simulink model "sgMdl_IO682_ARINC429Loopback"  (R2024b)
settings: Solver=FixedStepAuto  StartTime=0.0  StopTime=inf  RelTol=1e-3  EnableMultiTasking=on
undefined symbols (not defined in the file): IO682
libraries: speedgoatlib_IO682 x9
Description:
  | IO682 - ARINC 429 Loopback
settings Model: ModifiedByFormat=Speedgoat  SimulationMode=external  ExtModeTrigDuration=100000  Creator=Speedgoat  LastModifiedBy=Speedgoat
settings SolverCC: ConcurrentTasks=on  AlgebraicLoopSolver=TrustRegion  PositivePriorityOrder=on
settings DataIOCC: LimitDataPoints=on  SaveFormat=Array  ReturnWorkspaceOutputs=off
settings OptimizationCC: BlockReduction=off  OptimizeBlockIOStorage=off  BufferReuse=off  GlobalBufferReuse=off  ExpressionFolding=off  LocalBlockOutputs=off  OptimizeDataStoreBuffers=off  BusAssignmentInplaceUpdate=off
settings DebuggingCC: SolverPrmCheckMsg=warning  TasksWithSamePriorityMsg=none  UnconnectedInputMsg=warning  UnconnectedOutputMsg=warning  UnconnectedLineMsg=warning  AllowSymbolicDim=off  SFUnexpectedBacktrackingDiag=warning  SFNoUnconditionalDefaultTransitionDiag=warning  SFExecutionAtInitializationDiag=none  ArithmeticOperatorsInVariantConditions=warning
settings HardwareCC: ProdBitPerLong=64  ProdLongLongMode=on  ProdHWDeviceType=Intel->x86-64 (Linux 64)
settings ModelReferenceCC: EnableRefExpFcnMdlSchedulingChecks=on  PropagateSignalLabelsOutOfModel=off
settings SFSimCC: SimUseLocalCustomCode=off  CustomCodeUndefinedFunction=UseInterfaceOnly
settings RTWCC: Description=Speedgoat Real-Time Target Machine  SystemTargetFile=speedgoat.tlc  TemplateMakefile=slrealtime_default_tmf  RTWUseLocalCustomCode=off  Toolchain=Simulink Real-Time Toolchain  BuildConfiguration=Faster Runs  TargetLang=C++  GPUComputeCapability=3.5  DLArmComputeVersion=19.05
settings CodeAppCC: StateflowObjectComments=on
settings SimulinkRealTimeTargetCC: SubcomponentCodeInterfacePackaging=Reusable function  InstructionSetFMA=off  LogToMDFFile=off  SLRTFileLogMaxRuns=10  UseGCCFastMath=on
settings ConfigComp: CovMetricSettings=dw  CovSaveCumulativeToWorkspaceVar=on  CovSaveSingleToWorkspaceVar=on  CovExternalEMLEnable=off  CovSFcnEnable=off  CovBoundaryAbsTol=1.0e-5

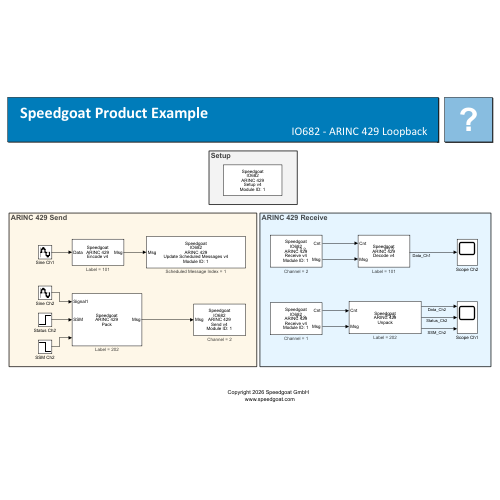
[thumbnail: Simulink's stored preview of the top-level diagram]
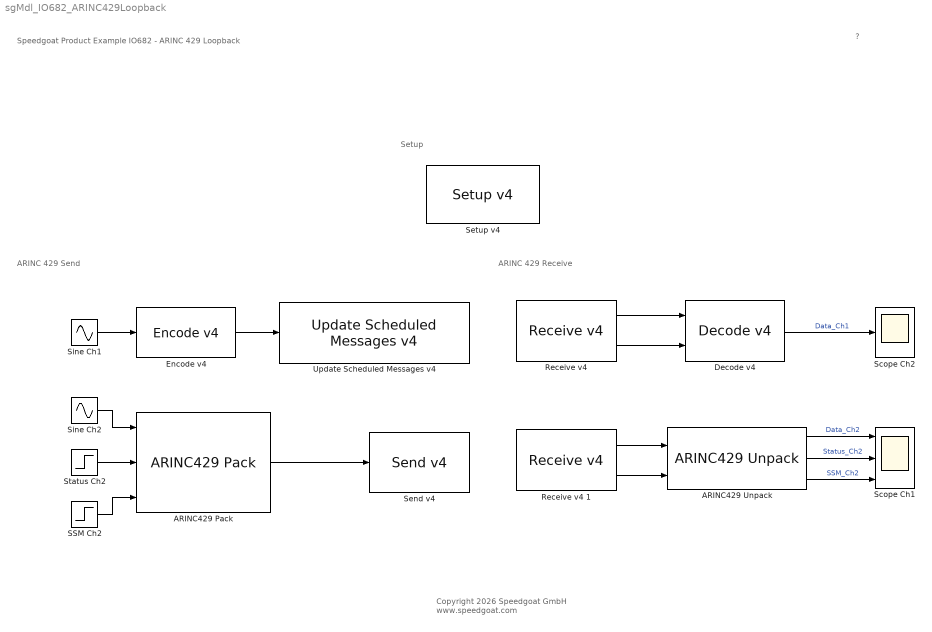
== system sgMdl_IO682_ARINC429Loopback ==
  note: ARINC 429 Send
  note: ARINC 429 Receive
  note: Setup
  note: Speedgoat Product Example
      | IO682 - ARINC 429 Loopback
  note: ?
  note: Copyright 2026 Speedgoat GmbH
      |  www.speedgoat.com
  "ARINC429 Pack " : speedgoatlib_IO682/ARINC429 Pack   parLabel=202  parSdi=2  parSsm=3  parSignals={ 'Sine', '11', '18', 'BNR', '10', '0', '-Inf', 'Inf', 'on'; 'Status Bit', '29', '1', 'DSC', '1', '0', '-Inf', 'Inf', 'off'; 'SSM', '30', '2', 'SSM', '1', '0', '-Inf', 'Inf', 'off' }
      settings: AttributesFormatString=Label = %<parLabel>  SourceProductName=IO682
  "ARINC429 Unpack " : speedgoatlib_IO682/ARINC429 Unpack   parLabel=202  parSdi=2  parSignals={ 'Sine', '11', '18', 'BNR', '10', '0', '-Inf', 'Inf', 'on'; 'Status Bit', '29', '1', 'DSC', '1', '0', '-Inf', 'Inf', 'off'; 'SSM', '30', '2', 'SSM', '1', '0', '-Inf', 'Inf', 'off' }  parEnTimeTag=off  parEnStatus=off  parEnRaw=off
      settings: AttributesFormatString=Label = %<parLabel>  SourceProductName=IO682
  "Decode v4 " : speedgoatlib_IO682/Decode v4   parLabel=101  parDataType=BNR  parResolution=10  parSdi=-1  parEnSDIBits=off  parHoldLastVal=on  parLabelOutput=off  parSSMOutput=off  parTimeTags=off  parStatus=off
      settings: AttributesFormatString=Label = %<parLabel>  SourceProductName=IO682
  "Encode v4 " : speedgoatlib_IO682/Encode v4   parLabel=101  parDataType=BNR  parResolution=10  parBits=19  parSdi=-1  parSsm=3  parEnSDIBits=off  parEnSSM=off
      settings: AttributesFormatString=Label = %<parLabel>  SourceProductName=IO682
  "Receive v4 " : speedgoatlib_IO682/Receive v4   parModuleId=1  parChannel=2  parMaxWords=50  parSampleTime=0.05  parEnTimeTags=off
      settings: AttributesFormatString=Channel = %<parChannel>  SourceProductName=IO682
  Receive v4 1 : speedgoatlib_IO682/Receive v4   parModuleId=1  parChannel=1  parMaxWords=50  parSampleTime=0.005  parEnTimeTags=off
      settings: AttributesFormatString=Channel = %<parChannel>  SourceProductName=IO682
  SSM Ch2 : Step  Time=5  Before=3  After=0  SampleTime=0
  Scope Ch1 : Scope  NumInputPorts=3
  Scope Ch2 : Scope
  "Send v4 " : speedgoatlib_IO682/Send v4   parModuleId=1  parChannel=2  parSampleTime=-1  parTxCtrl=off
      settings: AttributesFormatString=Channel = %<parChannel>  SourceProductName=IO682
  "Setup v4 " : speedgoatlib_IO682/Setup v4   parModuleId=1  parBoardVariant=IO682-8-8  parPciSlot=-1  parChannelMode=Manual  parInBitRate1=100000  parInBufferMode1=Individual  parInEnable1=on  parInParity1=on  parInInternalWrap1=off  parInBitRate2=100000  parInBufferMode2=Individual  parInEnable2=on  parInParity2=on  parInInternalWrap2=off  parInBitRate3=100000  parInBufferMode3=Individual  parInEnable3=on  parInParity3=on  parInInternalWrap3=off  parInBitRate4=100000  parInBufferMode4=Individual  parInEnable4=on  parInParity4=on  parInInternalWrap4=off  parInBitRate5=100000  parInBufferMode5=Individual  parInEnable5=off  parInParity5=on  parInInternalWrap5=off  parInBitRate6=100000  parInBufferMode6=Individual  parInEnable6=off  parInParity6=on  parInInternalWrap6=off  parInBitRate7=100000  parInBufferMode7=Individual  parInEnable7=off  parInParity7=on  parInInternalWrap7=off  parInBitRate8=100000  parInBufferMode8=Individual  parInEnable8=off  parInParity8=on  parInInternalWrap8=off  parInBitRate9=100000  parInBufferMode9=Individual  parInEnable9=on  parInParity9=on  parInInternalWrap9=off  parInBitRate10=100000  parInBufferMode10=Individual  parInEnable10=on  parInParity10=on  parInInternalWrap10=off  parInBitRate11=100000  parInBufferMode11=Individual  parInEnable11=on  parInParity11=on  parInInternalWrap11=off  parInBitRate12=100000  parInBufferMode12=Individual  parInEnable12=on  parInParity12=on  parInInternalWrap12=off  parInBitRate13=100000  parInBufferMode13=Individual  parInEnable13=on  parInParity13=on  parInInternalWrap13=off  parInBitRate14=100000  parInBufferMode14=Individual  parInEnable14=on  parInParity14=on  parInInternalWrap14=off  parInBitRate15=100000  parInBufferMode15=Individual  parInEnable15=on  parInParity15=on  parInInternalWrap15=off  parInBitRate16=100000  parInBufferMode16=Individual  parInEnable16=on  parInParity16=on  parInInternalWrap16=off  parOutBitRate1=100000  parOutParity1=Odd  parOutProtocolError1=None  parOutEnable1=on  parOutBitRate2=100000  parOutParity2=Odd  parOutProtocolError2=None  parOutEnable2=on  parOutBitRate3=100000  parOutParity3=Odd  parOutProtocolError3=None  parOutEnable3=on  parOutBitRate4=100000  parOutParity4=Odd  parOutProtocolError4=None  parOutEnable4=on  parOutBitRate5=100000  parOutParity5=Odd  parOutProtocolError5=None  parOutEnable5=off  parOutBitRate6=100000  parOutParity6=Odd  parOutProtocolError6=None  parOutEnable6=off  parOutBitRate7=100000  parOutParity7=Odd  parOutProtocolError7=None  parOutEnable7=off  parOutBitRate8=100000  parOutParity8=Odd  parOutProtocolError8=None  parOutEnable8=off  parOutBitRate9=100000  parOutParity9=Odd  parOutProtocolError9=None  parOutEnable9=on  parOutBitRate10=100000  parOutParity10=Odd  parOutProtocolError10=None  parOutEnable10=on  parOutBitRate11=100000  parOutParity11=Odd  parOutProtocolError11=None  parOutEnable11=on  parOutBitRate12=100000  parOutParity12=Odd  parOutProtocolError12=None  parOutEnable12=on  parOutBitRate13=100000  parOutParity13=Odd  parOutProtocolError13=None  parOutEnable13=on  parOutBitRate14=100000  parOutParity14=Odd  parOutProtocolError14=None  parOutEnable14=on  parOutBitRate15=100000  parOutParity15=Odd  parOutProtocolError15=None  parOutEnable15=on  parOutBitRate16=100000  parOutParity16=Odd  parOutProtocolError16=None  parOutEnable16=on  parChConfigFile=''  parScheduleMode=Manual  parScheduledMsgConfigFile=''  parHwDeviceId=hex2dec('0830')  parChInConfig=[158 8 7 7 1;158 8 7 7 1;158 8 7 7 1;158 8 7 7 1;158 8 8 7 1;158 8 8 7 1;158 8 8 7 1;158 8 8 7 1]  parChOutConfig=[158 0 4 7;158 0 4 7;158 0 4 7;158 0 4 7;158 0 4 8;158 0 4 8;158 0 4 8;158 0 4 8]  parScheduledMessages=[1 50 100 -1 1611137089]
      settings: SourceProductName=IO682
  Sine Ch1 : Sin  Amplitude=10  Frequency=2*pi  SampleTime=0.05
  Sine Ch2 : Sin  Amplitude=10  Frequency=2*pi  SampleTime=0.005
  Status Ch2 : Step  Time=3  SampleTime=0
  "Update Scheduled Messages v4 " : speedgoatlib_IO682/Update Scheduled Messages v4   parModuleId=1  parMessageId=1  parSampleTime=-1  parEnRate=off
      settings: AttributesFormatString=Scheduled Message Index = %<parMessageId>  SourceProductName=IO682
  wires:
  "Receive v4 "/1 -> "Decode v4 "/1
  "Decode v4 "/1 -> Scope Ch2/1  "Data_Ch1"
  "Encode v4 "/1 -> "Update Scheduled Messages v4 "/1
  Sine Ch1/1 -> "Encode v4 "/1
  "Receive v4 "/2 -> "Decode v4 "/2
  Sine Ch2/1 -> "ARINC429 Pack "/1
  "ARINC429 Pack "/1 -> "Send v4 "/1
  "ARINC429 Unpack "/1 -> Scope Ch1/1  "Data_Ch2"
  "ARINC429 Unpack "/2 -> Scope Ch1/2  "Status_Ch2"
  Status Ch2/1 -> "ARINC429 Pack "/2
  SSM Ch2/1 -> "ARINC429 Pack "/3
  "ARINC429 Unpack "/3 -> Scope Ch1/3  "SSM_Ch2"
  Receive v4 1/1 -> "ARINC429 Unpack "/1
  Receive v4 1/2 -> "ARINC429 Unpack "/2
